simulink model "furuta_clean"  (R2025b)
settings: Solver=VariableStepAuto  StartTime=0.0  StopTime=3  FixedStep=0.01  MaxStep=0.01  RelTol=1e-3
values from neighbouring files (symbols this model uses):
  Abig_s = [ A_s-B_s*K_s          , B_s*K_s ... (first row only)    [create_suspended_ctrl.m]    (also in simulink_companion.m)
  Ae = A_s - L_s * C_s    [create_suspended_ctrl.m]
  Ae_fi = fi( Ae_de, F_SIGNED, num_word, num_frac,      'RoundingMethod', rounding_method, 'OverflowAction', overflow_action )    [create_suspended_ctrl.m]
  Ae_fi_i = fi( Ae_de_i, F_SIGNED, num_word, num_frac,      'RoundingMethod', rounding_method, 'OverflowAction', overflow_action )    [create_inverted_ctrl_dt.m]
  Ae_i = A_i - L_i * C_i    [create_inverted_ctrl_dt.m]
  Be = [ B_s L_s ]    [create_suspended_ctrl.m]
  Be_fi = fi( Be_de, F_SIGNED, num_word, num_frac,      'RoundingMethod', rounding_method, 'OverflowAction', overflow_action )    [create_suspended_ctrl.m]
  Be_fi_i = fi( Be_de_i, F_SIGNED, num_word, num_frac,      'RoundingMethod', rounding_method, 'OverflowAction', overflow_action )    [create_inverted_ctrl_dt.m]
  Be_i = [ B_i L_i ]    [create_inverted_ctrl_dt.m]
  C = eye( 5, 5 )    [define_dynamics.m]
  C_i = [ 1 0 0 0 0 ... (first row only)    [create_inverted_ctrl.m]    (also in create_inverted_ctrl_dt.m; simulink_companion.m)
  C_s = [ 0 ]    [analyze_linear_dynamics.m]    (also in create_suspended_ctrl.m = [1 0 0 0 0; create_suspended_ctrl_dt.m = [ 1 0 0 0 0; simulink_companion.m = [ 1 0 0 0 0)
  Ce = eye(5)    [create_suspended_ctrl.m]
  Ce_fi = fi( Ce_de, F_SIGNED, num_word, num_frac,      'RoundingMethod', rounding_method, 'OverflowAction', overflow_action )    [create_suspended_ctrl.m]
  Ce_fi_i = fi( Ce_de_i, F_SIGNED, num_word, num_frac,      'RoundingMethod', rounding_method, 'OverflowAction', overflow_action )    [create_inverted_ctrl_dt.m]
  Ce_i = eye(5)    [create_inverted_ctrl_dt.m]
  De = zeros(5,4)    [create_suspended_ctrl.m]
  De_i = zeros(5,4)    [create_inverted_ctrl_dt.m]
  K_i = place( A_i, B_i, p )    [create_inverted_ctrl.m]    (also in create_inverted_ctrl_dt.m = zeros(size(K_i)); simulink_companion.m)
  K_s = place( A_s, B_s, p )    [analyze_linear_dynamics.m]    (also in create_suspended_ctrl.m = place( A_s, B_s, pc ); simulink_companion.m)
  T = 1/1000    (= 0.001)    [create_inverted_ctrl_dt.m]    (also in create_suspended_ctrl.m; system_identification_randin.m)
undefined symbols (not defined in the file or in its folder): Ae_de, Be_de, Ce_de
settings Model: Creator=shara  LastModifiedBy=shara

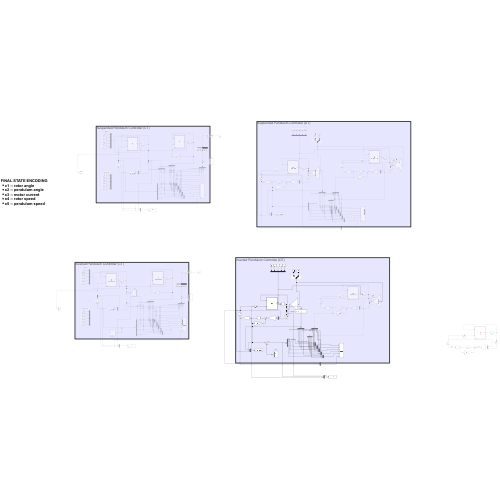
[thumbnail: Simulink's stored preview of the top-level diagram]
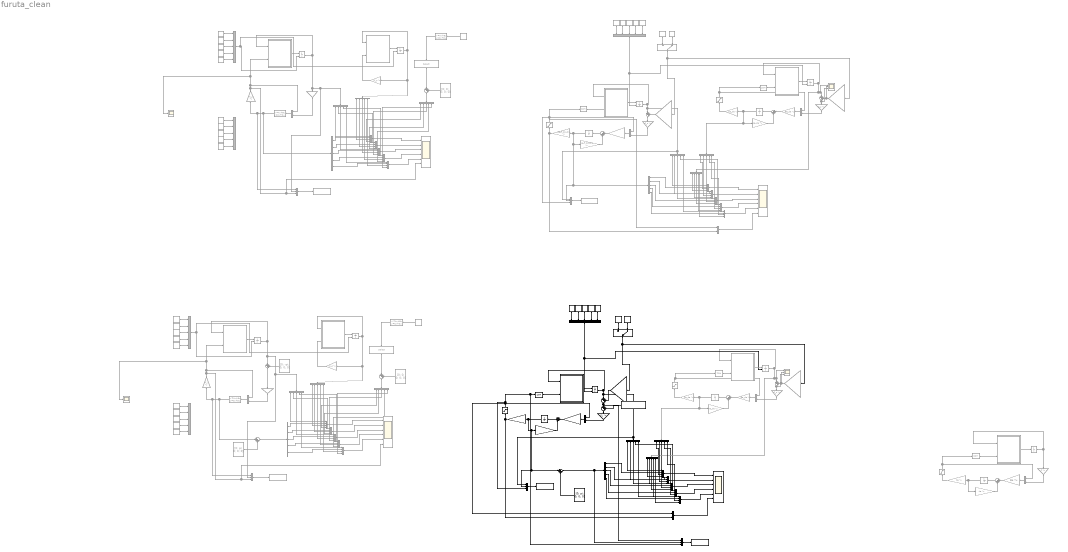
== system furuta_clean ==
  note: Suspended Pendulum Controller (DT)
  note: FINAL STATE ENCODING
      | x1 -- rotor angle
      | x2 -- pendulum angle
      | x3 -- motor current
      | x4 -- rotor speed
      | x5 -- pendulum speed
  note: Observer ICs
  note: Suspended Pendulum Controller (CT)
  note: State ICs
  note: Observer ICs
  note: Inverted Pendulum Controller (CT)
  note: Inverted Pendulum Controller (DT)
  note: State ICs
  Constant{1..4,6..10,58..61,63..67,87..90} (22 alike) : Constant  Commented=on  Value=0
  Constant11 : Constant  Value=pi-0.1
  Constant{12..15} (4 alike) : Constant  Value=0
  Constant5 : Constant  Commented=on  Value=pi-0.1
  Constant62 : Constant  Commented=on  Value=0.1
  Constant86 : Constant  Commented=on  Value=.1
  Demux{1..4,27..30,34..37} (12 alike) : Demux  Commented=on  Outputs=5
  Demux{5..8} (4 alike) : Demux  Outputs=5
  Gain1 : Gain  Commented=on  Gain=Be  Multiplication=Matrix(K*u)
  Gain10 : Gain  Commented=on  Gain=Be_de  Multiplication=Matrix(K*u)
  Gain11 : Gain  Commented=on  Gain=Ae_de  Multiplication=Matrix(K*u)
  Gain12 : Gain  Gain=Ce_fi_i.double  Multiplication=Matrix(K*u)
  Gain13 : Gain  Commented=on  Gain=Ce_de  Multiplication=Matrix(K*u)
  Gain{14,33,42..43} (4 alike) : Gain  Commented=on  Gain=C_s  Multiplication=Matrix(K*u)
  Gain15 : Gain  Gain=C_i  Multiplication=Matrix(K*u)
  Gain16 : Gain  Commented=on  Gain=[1;1;1;0;0]  Multiplication=Matrix(K*u)
  Gain17 : Gain  Gain=[1;1;1;0;0]  Multiplication=Matrix(K*u)
  Gain2 : Gain  Commented=on  Gain=Ae  Multiplication=Matrix(K*u)
  Gain27 : Gain  Commented=on  Gain=-K_s  Multiplication=Matrix(K*u)
  Gain3 : Gain  Commented=on  Gain=-K_i  Multiplication=Matrix(K*u)
  Gain32 : Gain  Commented=on  Gain=-K_s  Multiplication=Matrix(K*u)
  Gain36 : Gain  Commented=on  Gain=Be_fi.double  Multiplication=Matrix(K*u)
  Gain37 : Gain  Commented=on  Gain=Ae_fi.double  Multiplication=Matrix(K*u)
  Gain38 : Gain  Commented=on  Gain=Be_de  Multiplication=Matrix(K*u)
  Gain39 : Gain  Commented=on  Gain=Ae_de  Multiplication=Matrix(K*u)
  Gain4 : Gain  Commented=on  Gain=-K_s  Multiplication=Matrix(K*u)
  Gain40 : Gain  Commented=on  Gain=Ce_fi.double  Multiplication=Matrix(K*u)
  Gain41 : Gain  Commented=on  Gain=Ce_de  Multiplication=Matrix(K*u)
  Gain44 : Gain  Commented=on  Gain=[1;1;1;0;0]  Multiplication=Matrix(K*u)
  Gain45 : Gain  Commented=on  Gain=[1;1;1;0;0]  Multiplication=Matrix(K*u)
  Gain5 : Gain  Commented=on  Gain=Ce  Multiplication=Matrix(K*u)
  Gain6 : Gain  Commented=on  Gain=C_i  Multiplication=Matrix(K*u)
  Gain7 : Gain  Gain=Be_fi_i.double  Multiplication=Matrix(K*u)
  Gain8 : Gain  Commented=on  Gain=C  Multiplication=Matrix(K*u)
  Gain9 : Gain  Gain=Ae_fi_i.double  Multiplication=Matrix(K*u)
  Integrator{1,3..4,12..13,15..16} (7 alike) : Integrator  Commented=on  InitialConditionSource=external
  Integrator2 : Integrator  Commented=on
  Integrator5 : Integrator  InitialConditionSource=external
  MATLAB Function1 : MATLAB Function  Commented=on  TreatAsAtomicUnit=on
  MATLAB Function13 : MATLAB Function  Commented=on  TreatAsAtomicUnit=on
  MATLAB Function16 : MATLAB Function  Commented=on  TreatAsAtomicUnit=on
  MATLAB Function2 : MATLAB Function  Commented=on  TreatAsAtomicUnit=on
  MATLAB Function3 : MATLAB Function  TreatAsAtomicUnit=on
  MATLAB Function4 : MATLAB Function  Commented=on  TreatAsAtomicUnit=on
  MATLAB Function5 : MATLAB Function  Commented=on  TreatAsAtomicUnit=on
  MATLAB Function7 : MATLAB Function  Commented=on  TreatAsAtomicUnit=on
  MATLAB Function8 : MATLAB Function  Commented=on  TreatAsAtomicUnit=on
  Manual Switch1 : ManualSwitch  CurrentSetting=0
  Manual Switch3 : ManualSwitch  Commented=on  CurrentSetting=0
  Mux{,9..10,20,52,69..70} (7 alike) : Mux  Commented=on  Inputs=2
  Mux1 : Mux  Inputs=2
  Mux11 : Mux  Commented=on  Inputs=3
  Mux{12..14,16..17} (5 alike) : Mux
  Mux15 : Mux  Inputs=5
  Mux18 : Mux  Inputs=3
  Mux19 : Mux  Inputs=2
  Mux{2,6,45,49,65} (5 alike) : Mux  Commented=on  Inputs=5
  Mux21 : Mux  Inputs=3
  Mux{3..5,7..8,46..48,50..51,62..64,66..67} (15 alike) : Mux  Commented=on
  Mux53 : Mux  Commented=on  Inputs=3
  Mux68 : Mux  Commented=on  Inputs=3
  Random Number1 : RandomNumber  Commented=on  Variance=0.0001  SampleTime=0.001
  Random Number2 : RandomNumber  Variance=0.0001  SampleTime=0.001
  Saturation : Saturate  Commented=on  UpperLimit=4.8  LowerLimit=-4.8
  Saturation1 : Saturate  Commented=on  UpperLimit=12  LowerLimit=-12
  Saturation2 : Saturate  Commented=on  UpperLimit=4.8  LowerLimit=-4.8
  Saturation3 : Saturate  UpperLimit=4.8  LowerLimit=-4.8
  Saturation4 : Saturate  Commented=on  UpperLimit=12  LowerLimit=-12
  Scope1 : Scope  Commented=on
      settings: ActiveDisplayYMinimum=-1  ActiveDisplayYMaximum=1
  Scope11 : Scope  Commented=on
      settings: ActiveDisplayYMinimum=-1  ActiveDisplayYMaximum=1  DataLoggingVariableName=ScopeData11
  Scope14 : Scope  Commented=on  NumInputPorts=6
      settings: ActiveDisplayYMinimum=-0.016592743929513151  ActiveDisplayYMaximum=0.012821370046477933  DataLoggingVariableName=ScopeData14
  Scope16 : Scope  Commented=on  NumInputPorts=6
      settings: ActiveDisplayYMinimum=-0.10215866473662746  ActiveDisplayYMaximum=0.014796355106009663  DataLoggingVariableName=ScopeData16
  Scope17 : Scope  Commented=on  NumInputPorts=3
      settings: ActiveDisplayYMinimum=-5.519017462446989  ActiveDisplayYMaximum=7.2103752502822056  DataLoggingVariableName=ScopeData17
  Scope2 : Scope  Commented=on  NumInputPorts=6
      settings: ActiveDisplayYMinimum=-13.033331906556104  ActiveDisplayYMaximum=117.29980558762723
  Scope3 : Scope  NumInputPorts=6
      settings: ActiveDisplayYMinimum=-0.0095998444334833288  ActiveDisplayYMaximum=0.0099978590254368033  DataLoggingVariableName=ScopeData2
  Scope4 : Scope  Commented=on  NumInputPorts=3
      settings: ActiveDisplayYMinimum=-5.519017462446989  ActiveDisplayYMaximum=7.2103752502822056  DataLoggingVariableName=ScopeData3
  Selector1 : Selector  Commented=on  InputPortWidth=10  IndexOptions=Index vector (dialog)  Indices=[1:5]  OutputSizes=1
  Selector2 : Selector  Commented=on  InputPortWidth=10  IndexOptions=Index vector (dialog)  Indices=[1:5]  OutputSizes=1
  State-Space1 : StateSpace  Commented=on  A=Ae_i  B=Be_i  C=Ce_i  D=De_i  InitialCondition=[0 0.1 0 0 0]
  State-Space10 : StateSpace  Commented=on  A=Ae  B=Be  C=Ce  D=De  InitialCondition=[0 0.1 0 0 0]
  State-Space2 : StateSpace  Commented=on  A=Abig_s  B=zeros(10,1)  C=[ eye(5), zeros(5); zeros(5), zeros(5) ]  D=zeros(10,1)  InitialCondition=[0; 0.1; 0; 0; 0; 0; 0; 0; 0; 0]
  State-Space9 : StateSpace  Commented=on  A=Abig_s  B=zeros(10,1)  C=[ eye(5), zeros(5); zeros(5), zeros(5) ]  D=zeros(10,1)  InitialCondition=[0; 0.1; 0; 0; 0; 0; 0; 0; 0; 0]
  Sum{,1..2,4..5,7,13..17} (11 alike) : Sum  Commented=on  Inputs=|++
  Sum{3,6,8..9} (4 alike) : Sum  Inputs=|++
  To Workspace : ToWorkspace  Commented=on  VariableName=CTsim  SaveFormat=Timeseries  SampleTime=-1
  To Workspace1 : ToWorkspace  Commented=on  VariableName=CTsim1  SaveFormat=Timeseries  SampleTime=-1
  To Workspace2 : ToWorkspace  Commented=on  VariableName=DTsim  SaveFormat=Timeseries  SampleTime=-1
  To Workspace3 : ToWorkspace  VariableName=DTsim1  SaveFormat=Timeseries  SampleTime=-1
  To Workspace4 : ToWorkspace  VariableName=DTsimI  SaveFormat=Timeseries  SampleTime=-1
  Unit Delay1 : UnitDelay  Commented=on  InitialCondition=[0 0.1 0 0 0];  SampleTime=T  HasFrameUpgradeWarning=on
  Unit Delay2 : UnitDelay  InitialCondition=[0 0.1 0 0 0];  SampleTime=T  HasFrameUpgradeWarning=on
  Unit Delay3 : UnitDelay  Commented=on  InitialCondition=[0 0.1 0 0 0];  SampleTime=T  HasFrameUpgradeWarning=on
  Unit Delay4 : UnitDelay  Commented=on  InitialCondition=[0 0.01 0 0 0]  SampleTime=-1  HasFrameUpgradeWarning=on
  Unit Delay5 : UnitDelay  Commented=on  InitialCondition=[0 0.01 0 0 0]  SampleTime=-1  HasFrameUpgradeWarning=on
  Zero-Order Hold : ZeroOrderHold  Commented=on  SampleTime=T
  Zero-Order Hold1 : ZeroOrderHold  Commented=on  SampleTime=T
  Zero-Order Hold2 : ZeroOrderHold  SampleTime=T
  Zero-Order Hold3 : ZeroOrderHold  Commented=on  SampleTime=-1
  Zero-Order Hold5 : ZeroOrderHold  Commented=on  SampleTime=-1
  Zero1 : Constant  Commented=on  Value=0  OutDataTypeStr=Inherit: Inherit via back propagation
  Zero2 : Constant  Value=0  OutDataTypeStr=Inherit: Inherit via back propagation
  Zero5 : Constant  Commented=on  Value=0  OutDataTypeStr=Inherit: Inherit via back propagation
  Zero6 : Constant  Commented=on  Value=0  OutDataTypeStr=Inherit: Inherit via back propagation
  x_eq1 : Constant  Commented=on  Value=[0; 0; 0; 0; 0]  VectorParams1D=off
  x_eq2 : Constant  Commented=on  Value=[0; -pi; 0; 0; 0]  VectorParams1D=off
  x_eq3 : Constant  Commented=on  Value=[0; 0; 0; 0; 0]  VectorParams1D=off
  x_eq4 : Constant  Commented=on  Value=[0; pi; 0; 0; 0]  VectorParams1D=off
  x_eq5 : Constant  Value=[0; -pi; 0; 0; 0]
  x_eq6 : Constant  Value=[0; pi; 0; 0; 0]  VectorParams1D=off
  wires:
  Demux28/1 -> Mux46/1  "theta_1 (GROUND TRUTH)"
  Demux28/4 -> Mux50/1  "theta_1_d"
  Constant65/1 -> Mux49/5
  Mux51/1 -> Scope14/3
  Demux27/4 -> Mux50/2  "theta_1_dot"
  MATLAB Function7/1(dx) -> Integrator12/1
  Constant58/1 -> Mux45/3
  Mux50/1 -> Scope14/4
  Mux48/1 -> Scope14/5
  Mux47/1 -> Scope14/2
  Constant59/1 -> Mux45/4
  Demux27/1 -> Mux46/2  "theta_1"
  Constant66/1 -> Mux49/1
  Constant64/1 -> Mux49/4
  Constant62/1 -> Mux49/2
  Constant67/1 -> Mux45/2
  Integrator12/1 -> Mux53/2, Demux28/1, Gain33/1, MATLAB Function7/1(x)
  Mux46/1 -> Scope14/1
  Demux27/2 -> Mux47/2  "theta_2"
  Constant60/1 -> Mux45/5
  Demux28/3 -> Mux51/1  "i"
  Gain33/1 -> Mux52/2
  Demux27/3 -> Mux51/2  "i"
  Demux28/2 -> Mux47/1  "theta_2"
  Demux28/5 -> Mux48/1  "theta_2_dot"
  Constant61/1 -> Mux45/1
  Demux27/5 -> Mux48/2  "theta_2_dot"
  Mux49/1 -> Integrator13/2, Integrator12/2
  Constant63/1 -> Mux49/3
  State-Space10/1 -> Demux27/1, Mux53/1, Gain27/1
  Gain27/1 -> Scope14/6, Mux53/3, Mux52/1, Scope11/1, MATLAB Function7/2(V)
  Mux52/1 -> State-Space10/1
  MATLAB Function8/1(dx) -> Integrator13/1
  Integrator13/1 -> Demux29/1, Gain32/1, MATLAB Function8/1(x)
  Gain32/1 -> MATLAB Function8/2(V)
  Demux29/1 -> Mux46/3  "theta_1 (GROUND TRUTH)"
  Demux29/2 -> Mux47/3  "theta_2"
  Demux29/3 -> Mux51/3  "i"
  Demux29/4 -> Mux50/3  "theta_1_d"
  Demux29/5 -> Mux48/3  "theta_2_dot"
  x_eq3/1 -> Sum13/2
  Zero5/1 -> State-Space9/1
  Selector1/1 -> Sum13/1
  State-Space9/1 -> Selector1/1
  Sum13/1 -> Demux30/1
  Demux30/1 -> Mux46/4  "theta_1 (GROUND TRUTH)"
  Demux30/2 -> Mux47/4  "theta_2"
  Demux30/3 -> Mux51/4  "i"
  Demux30/4 -> Mux50/4  "theta_1_d"
  Demux30/5 -> Mux48/4  "theta_2_dot"
  Mux53/1 -> To Workspace/1
  Demux37/4 -> Mux66/4
  Demux37/1 -> Mux62/4  "theta_1 (GT, double estimator)"
  Demux37/2 -> Mux63/4
  Demux37/3 -> Mux67/4
  Demux34/2 -> Mux63/3  "theta_2"
  Mux66/1 -> Scope16/4
  Demux35/4 -> Mux66/2
  Demux36/3 -> Mux67/1  "i"
  Constant86/1 -> Mux65/2
  Demux37/5 -> Mux64/4
  Constant88/1 -> Mux65/4
  Demux35/2 -> Mux63/2
  Mux64/1 -> Scope16/5
  Demux35/3 -> Mux67/2
  Demux34/4 -> Mux66/3  "theta_1_d"
  Constant87/1 -> Mux65/3
  Demux35/5 -> Mux64/2
  Demux36/2 -> Mux63/1  "theta_2"
  Mux63/1 -> Scope16/2
  Demux36/5 -> Mux64/1  "theta_2_dot"
  Mux62/1 -> Scope16/1
  Demux36/1 -> Mux62/1  "theta_1 (GT, fi estimator))"
  Mux67/1 -> Scope16/3
  Integrator16/1 -> MATLAB Function16/1(x), Sum17/1, Mux68/1, Demux36/1
  Demux34/5 -> Mux64/3  "theta_2_dot"
  Demux34/3 -> Mux67/3  "i"
  MATLAB Function16/1(dx) -> Integrator16/1
  Demux36/4 -> Mux66/1  "theta_1_d"
  Mux65/1 -> Integrator15/2, Integrator16/2
  Constant90/1 -> Mux65/1
  Demux35/1 -> Mux62/2  "theta_1 (fi estimator)"
  Demux34/1 -> Mux62/3  "theta1 (double estimator)"
  Constant89/1 -> Mux65/5
  Gain36/1 -> Sum14/1
  Gain37/1 -> Sum14/2
  Sum14/1 -> Unit Delay3/1
  Unit Delay3/1 -> Demux35/1, Mux68/2, Gain37/1, Gain40/1
  Mux69/1 -> Gain36/1
  Gain40/1 -> Saturation/1, Mux/2
  Unit Delay4/1 -> Demux34/1, Gain39/1, Gain41/1
  Gain38/1 -> Sum15/1
  Sum15/1 -> Unit Delay4/1
  Gain41/1 -> Saturation1/1
  Mux70/1 -> Gain38/1
  Zero-Order Hold5/1 -> MATLAB Function13/2(V)
  MATLAB Function13/1(dx) -> Integrator15/1
  Gain39/1 -> Sum15/2
  Integrator15/1 -> MATLAB Function13/1(x), Scope17/1, Sum16/1, Demux37/1
  Gain43/1 -> Mux69/2
  Sum16/1 -> Scope17/3, Gain42/1
  Gain42/1 -> Mux70/2
  Gain44/1 -> Scope17/2, Sum16/2
  Gain45/1 -> Sum17/2
  Sum17/1 -> Gain43/1
  Zero6/1 -> Manual Switch3/2
  Random Number1/1 -> Manual Switch3/1
  Manual Switch3/1 -> Gain44/1, Gain45/1
  Saturation/1 -> Zero-Order Hold/1, Mux68/3, Mux/1, Mux69/1
  Saturation1/1 -> Zero-Order Hold5/1, Mux70/1
  Mux68/1 -> To Workspace2/1
  Mux/1 -> Scope16/6
  Zero-Order Hold/1 -> MATLAB Function16/2(V)
  Mux9/1 -> Gain1/1
  MATLAB Function2/1(dx) -> Integrator2/1
  Gain8/1 -> Mux9/2
  Sum1/1 -> Unit Delay1/1
  Gain2/1 -> Sum1/2
  Gain5/1 -> Saturation2/1
  Integrator2/1 -> Gain8/1, MATLAB Function2/1(x)
  Gain1/1 -> Sum1/1
  Zero-Order Hold1/1 -> MATLAB Function2/2(V)
  Unit Delay1/1 -> Gain2/1, Gain5/1
  Saturation2/1 -> Zero-Order Hold1/1, Mux9/1
  Unit Delay5/1 -> Demux5/1, Gain11/1, Gain13/1
  MATLAB Function5/1(dx) -> Integrator3/1
  Demux3/1 -> Mux3/3  "theta_1 (GROUND TRUTH)"
  Demux2/1 -> Mux3/1  "theta_1 (GROUND TRUTH)"
  Gain11/1 -> Sum4/2
  Mux20/1 -> Gain10/1
  Sum2/1 -> Demux4/1
  Demux5/1 -> Mux12/3  "theta1 (double estimator)"
  x_eq1/1 -> Sum2/2
  Saturation4/1 -> Zero-Order Hold3/1, Mux20/1
  Demux3/5 -> Mux5/3  "theta_2_dot"
  Demux3/4 -> Mux7/3  "theta_1_d"
  Constant2/1 -> Mux2/4
  Demux1/5 -> Mux5/2  "theta_2_dot"
  Constant14/1 -> Mux15/5
  Constant15/1 -> Mux15/1
  Mux17/1 -> Scope3/3
  Manual Switch1/1 -> Gain16/1, Gain17/1
  Mux19/1 -> Gain7/1
  Demux1/1 -> Mux3/2  "theta_1"
  Demux5/4 -> Mux16/3  "theta_1_d"
  Gain4/1 -> MATLAB Function5/2(V)
  Constant4/1 -> Mux2/1
  Demux1/2 -> Mux4/2  "theta_2"
  Random Number2/1 -> Manual Switch1/1
  Sum4/1 -> Unit Delay5/1
  Mux6/1 -> Integrator3/2, Integrator1/2
  Constant10/1 -> Mux2/2
  Demux4/1 -> Mux3/4  "theta_1 (GROUND TRUTH)"
  Sum3/1 -> Unit Delay2/1
  Demux1/3 -> Mux8/2  "i"
  Demux6/1 -> Mux12/2  "theta_1 (fi estimator)"
  State-Space2/1 -> Selector2/1
  Constant9/1 -> Mux6/1
  Demux5/3 -> Mux17/3  "i"
  Demux6/5 -> Mux14/2
  Constant11/1 -> Mux15/2
  Gain16/1 -> Scope4/2, Sum5/2
  Constant12/1 -> Mux15/3
  Zero-Order Hold3/1 -> MATLAB Function1/2(V)
  Demux7/1 -> Mux12/1  "theta_1 (GT, fi estimator))"
  Gain10/1 -> Sum4/1
  Demux8/5 -> Mux14/4
  Demux7/4 -> Mux16/1  "theta_1_d"
  Demux1/4 -> Mux7/2  "theta_1_dot"
  Demux2/3 -> Mux8/1  "i"
  Mux10/1 -> State-Space1/1
  Demux7/5 -> Mux14/1  "theta_2_dot"
  Gain7/1 -> Sum3/1
  Mux12/1 -> Scope3/1
  Mux7/1 -> Scope2/4
  Demux7/3 -> Mux17/1  "i"
  Mux3/1 -> Scope2/1
  Mux14/1 -> Scope3/5
  Gain14/1 -> Mux20/2
  Zero1/1 -> State-Space2/1
  Integrator1/1 -> Sum/1, Mux11/2, Demux2/1, MATLAB Function4/1(x)
  Demux2/2 -> Mux4/1  "theta_2"
  Gain13/1 -> Saturation4/1
  Sum5/1 -> Scope4/3, Gain14/1
  Gain12/1 -> Saturation3/1, Mux1/2
  Demux4/5 -> Mux5/4  "theta_2_dot"
  Integrator4/1 -> MATLAB Function1/1(x), Scope4/1, Sum5/1, Demux8/1
  Demux6/4 -> Mux16/2
  Demux8/1 -> Mux12/4  "theta_1 (GT, double estimator)"
  Unit Delay2/1 -> Sum9/1, Mux18/2, Gain9/1, Gain12/1
  Mux1/1 -> Scope3/6
  Gain15/1 -> Mux19/2
  Demux8/2 -> Mux13/4
  State-Space1/1 -> Sum7/1, Mux11/1, Gain3/1
  Constant13/1 -> Mux15/4
  Gain9/1 -> Sum3/2
  Demux2/5 -> Mux5/1  "theta_2_dot"
  Integrator3/1 -> Demux3/1, Gain4/1, MATLAB Function5/1(x)
  Constant6/1 -> Mux6/3
  Mux13/1 -> Scope3/2
  Demux4/4 -> Mux7/4  "theta_1_d"
  Demux5/5 -> Mux14/3  "theta_2_dot"
  Constant1/1 -> Mux2/3
  MATLAB Function3/1(dx) -> Integrator5/1
  Demux6/3 -> Mux17/2
  Demux8/4 -> Mux16/4
  Demux4/2 -> Mux4/4  "theta_2"
  Sum6/1 -> Mux21/1, Sum8/1
  Mux15/1 -> Integrator4/2, Integrator5/2
  Demux7/2 -> Mux13/1  "theta_2"
  Constant8/1 -> Mux6/5
  Demux3/3 -> Mux8/3  "i"
  Demux4/3 -> Mux8/4  "i"
  MATLAB Function4/1(dx) -> Integrator1/1
  MATLAB Function1/1(dx) -> Integrator4/1
  Demux3/2 -> Mux4/3  "theta_2"
  Constant7/1 -> Mux6/4
  Gain6/1 -> Mux10/2
  Zero-Order Hold2/1 -> MATLAB Function3/2(V)
  Demux2/4 -> Mux7/1  "theta_1_d"
  Demux5/2 -> Mux13/3  "theta_2"
  Zero2/1 -> Manual Switch1/2
  Demux8/3 -> Mux17/4
  Mux4/1 -> Scope2/2
  Mux5/1 -> Scope2/5
  Selector2/1 -> Sum2/1
  Mux11/1 -> To Workspace1/1
  Constant3/1 -> Mux2/5
  Gain17/1 -> Sum6/2
  Mux16/1 -> Scope3/4
  Integrator5/1 -> MATLAB Function3/1(x), Sum6/1, Mux18/1, Demux7/1
  Gain3/1 -> Scope2/6, Mux11/3, Mux10/1, Scope1/1, MATLAB Function4/2(V)
  Saturation3/1 -> Mux21/3, Zero-Order Hold2/1, Mux18/3, Mux19/1, Mux1/1
  Mux8/1 -> Scope2/3
  Mux18/1 -> To Workspace3/1
  Constant5/1 -> Mux6/2
  Demux6/2 -> Mux13/2
  Sum/1 -> Gain6/1
  x_eq2/1 -> Sum/2
  Sum7/1 -> Demux1/1
  x_eq4/1 -> Sum7/2
  Sum8/1 -> Gain15/1
  x_eq5/1 -> Sum8/2
  x_eq6/1 -> Sum9/2
  Sum9/1 -> Mux21/2, Demux6/1
  Mux21/1 -> To Workspace4/1

== matlab function furuta_clean/MATLAB Function1 ==
  data: x input; dx output; V input
function dx = nonlinear_furuta(x, V)

dx = simulate_dynamics_func( x, V );

== matlab function furuta_clean/MATLAB Function2 ==
  data: x input; dx output; V input
function dx = nonlinear_furuta(x, V)

dx = simulate_dynamics_func( x, V );

== matlab function furuta_clean/MATLAB Function3 ==
  data: x input; dx output; V input
function dx = nonlinear_furuta(x, V)

dx = simulate_dynamics_func( x, V );

== matlab function furuta_clean/MATLAB Function4 ==
  data: x input; dx output; V input
function dx = nonlinear_furuta(x, V)

dx = simulate_dynamics_func( x, V );

== matlab function furuta_clean/MATLAB Function5 ==
  data: x input; dx output; V input
function dx = nonlinear_furuta(x, V)

dx = simulate_dynamics_func( x, V );

== matlab function furuta_clean/MATLAB Function7 ==
  data: x input; dx output; V input
function dx = nonlinear_furuta(x, V)

dx = simulate_dynamics_func( x, V );

== matlab function furuta_clean/MATLAB Function8 ==
  data: x input; dx output; V input
function dx = nonlinear_furuta(x, V)

dx = simulate_dynamics_func( x, V );

== matlab function furuta_clean/MATLAB Function13 ==
  data: x input; dx output; V input
function dx = nonlinear_furuta(x, V)

dx = simulate_dynamics_func( x, V );

== matlab function furuta_clean/MATLAB Function16 ==
  data: x input; dx output; V input
function dx = nonlinear_furuta(x, V)

dx = simulate_dynamics_func( x, V );
